simulink model "droneCorke"  (R2018a)
settings: Solver=VariableStepAuto  StartTime=0.0  StopTime=10.0  RelTol=1e-3
values from neighbouring files (symbols this model uses):
  MapMatrix = diag([ 1, -1, -1, -1, -1, 1, 1, -1, -1, -1, -1, 1])    [droneCorkeInit.m]
undefined symbols (not defined in the file or in its folder): Cofficients, quadrotor
libraries: simulink x14, roblocks x2
settings Model: Creator=dinies33  LastModifiedBy=dinies33

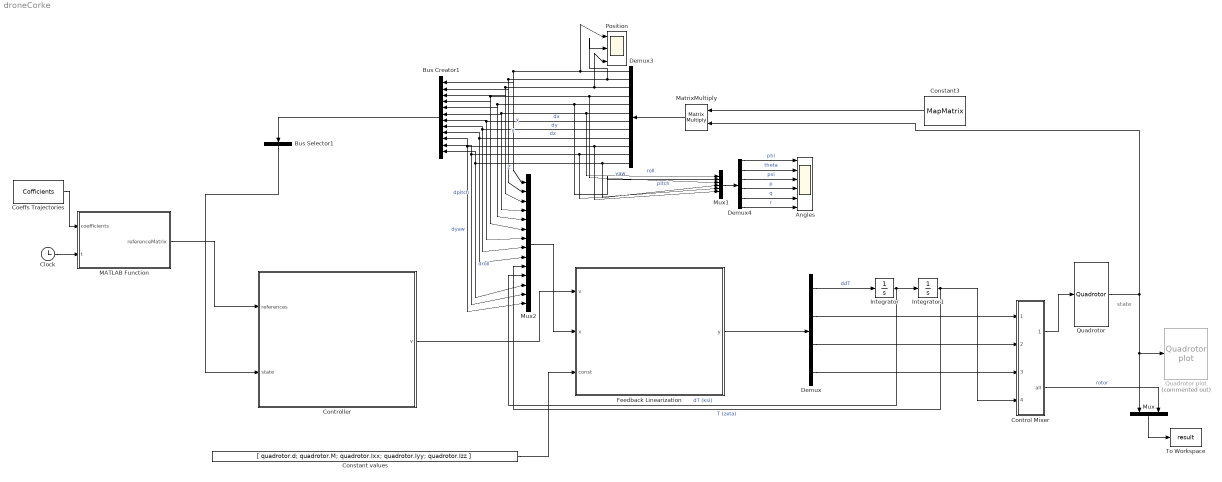
== system droneCorke ==
  note: state
  Angles : Scope  NumInputPorts=6
  Bus Creator1 : BusCreator  Inputs='X','Y','Z','yaw','pitch','roll','dx','dy','dz','dyaw','dpitch','droll'
  Bus Selector1 : BusSelector  OutputSignals=X,Y,Z,dx,dy,dz,yaw,dyaw  OutputAsBus=on
  Clock : Clock
  Coeffs Trajectories : Constant  Value=Cofficients
  Constant values : Constant  Value=[ quadrotor.d; quadrotor.M; quadrotor.Ixx; quadrotor.Iyy; quadrotor.Izz ]
  Constant3 : Constant  Value=MapMatrix
  Control Mixer : Subsystem  AncestorBlock=roblocks/Vehicles/Control Mixer 4  mask{quad=quadrotor, maxrot=1000, minrot=5}
      mask prompts: quad "Quadrotor parameters"; maxrot "Maximum rotor speed (rad/s)"; minrot "Minimum rotor speed (rad/s)"
      mask help: Quadrotor control mixer
      mask Help:
      | Determine rotor speeds based on desired torques and thrust, and propellor model
      | 
      | <b>Inputs::</b>
      | tau<sub>x</sub> (1x1)    desired rolling torque [Nm]
      | 
      | tau<sub>y</sub> (1x1)    desired pitching torque [Nm]
      | tau<sub>z</sub> (1x1)    desired yawing torque [Nm]
      | T (1x1)          desired thrust [N]
      | 
      | <b>Outputs::</b>
      | 
      | w1 (1x1) angular velocity of rotor 1 [rad]
      | w2 (1x1) angular velocity of rotor 2 [rad]
      | w3 (1x1) angular velocity of rotor 3 [rad]
      | w4 (1x1) angular velocity of rotor 4 [rad]
      | 
      | <b>Notes::</b>
      | 
      | - Assumes the rotor labelling convention of RVC Fig 4.16.
      | - The quadrotor is underactuated and has only 4 inputs.
      mask Display:
      | port_label('output',1,'\varpi','texmode','on');
      | port_label('output',2,'\tau_a','texmode','on');
      | port_label('input',1,'\tau_x','texmode','on');
      | port_label('input',2,'\tau_y','texmode','on');
      | port_label('input',3,'\tau_z','texmode','on');
      | port_label('input',4,'T','texmode','on');
  Controller : Subsystem
  Demux : Demux
  Demux3 : Demux  Outputs=12
  Demux4 : Demux  Outputs=6
  Feedback Linearization : MATLAB Function  TreatAsAtomicUnit=on
  Integrator : Integrator
  Integrator1 : Integrator
  MATLAB Function : MATLAB Function  TreatAsAtomicUnit=on
  MatrixMultiply : Product  Multiplication=Matrix(*)
  Mux : Mux  Inputs=2
  Mux1 : Mux  Inputs=6
  Mux2 : Mux  Inputs=14
  Position : Scope  NumInputPorts=3
  Quadrotor : roblocks/Vehicles/Quadrotor  quad=quadrotor  x0=[0 0 -5]  groundflag=on
      link override Dynamics: FunctionName=corke_dynamics
  Quadrotor plot : roblocks/Vehicles/Quadrotor plot  Commented=on  quad=quadrotor  xydim=2  zdim=10
      link override Plotter: FunctionName=corke_plot  Parameters=[xydim, zdim], 1, 1,quad
  To Workspace : ToWorkspace  VariableName=result  SampleTime=-1
  wires:
  Control Mixer/1(omega) -> Quadrotor/1
  Control Mixer/2(all) -> Mux/2  "rotor"
  Demux/2 -> Control Mixer/1(tau roll)
  Mux/1 -> To Workspace/1
  Demux/3 -> Control Mixer/2(tau pitch)
  Demux/4 -> Control Mixer/3(tau yaw)
  Bus Creator1/1 -> Bus Selector1/1
  Demux3/7 -> Mux2/7, Bus Creator1/7  "dx"
  Constant3/1 -> MatrixMultiply/1
  Demux3/10 -> Mux1/6, Mux2/14, Bus Creator1/10  "dyaw"
  Demux3/5 -> Mux1/2, Mux2/5, Bus Creator1/5  "pitch"
  Quadrotor/1 -> MatrixMultiply/2, Quadrotor plot/1, Mux/1
  Demux3/11 -> Mux1/5, Mux2/13, Bus Creator1/11  "dpitch"
  Demux3/9 -> Mux2/9, Bus Creator1/9  "dz"
  Demux3/12 -> Mux1/4, Mux2/12, Bus Creator1/12  "droll"
  Demux3/3 -> Position/3, Mux2/3, Bus Creator1/3  "Z"
  Demux3/4 -> Mux1/3, Mux2/6, Bus Creator1/4  "yaw"
  Demux3/8 -> Mux2/8, Bus Creator1/8  "dy"
  MatrixMultiply/1 -> Demux3/1
  Demux3/2 -> Position/2, Mux2/2, Bus Creator1/2  "Y"
  Demux3/6 -> Mux2/4, Bus Creator1/6, Mux1/1  "roll"
  Demux4/1 -> Angles/1  "phi"
  Demux4/4 -> Angles/4  "p"
  Demux4/3 -> Angles/3  "psi"
  Demux4/2 -> Angles/2  "theta"
  Demux4/5 -> Angles/5  "q"
  Demux4/6 -> Angles/6  "r"
  Mux1/1 -> Demux4/1
  Demux3/1 -> Position/1, Mux2/1, Bus Creator1/1  "X"
  Constant values/1 -> Feedback Linearization/3(const)
  Feedback Linearization/1(y) -> Demux/1
  Demux/1 -> Integrator/1  "ddT"
  Integrator/1 -> Mux2/11, Integrator1/1  "dT (ksi)"
  Integrator1/1 -> Mux2/10, Control Mixer/4(total thrust)  "T (zeta)"
  Mux2/1 -> Feedback Linearization/2(x)
  Controller/1(v) -> Feedback Linearization/1(v)
  MATLAB Function/1(referenceMatrix) -> Controller/1(references)
  Clock/1 -> MATLAB Function/2(t)
  Coeffs Trajectories/1 -> MATLAB Function/1(coefficients)
  Bus Selector1/1 -> Controller/2(state)

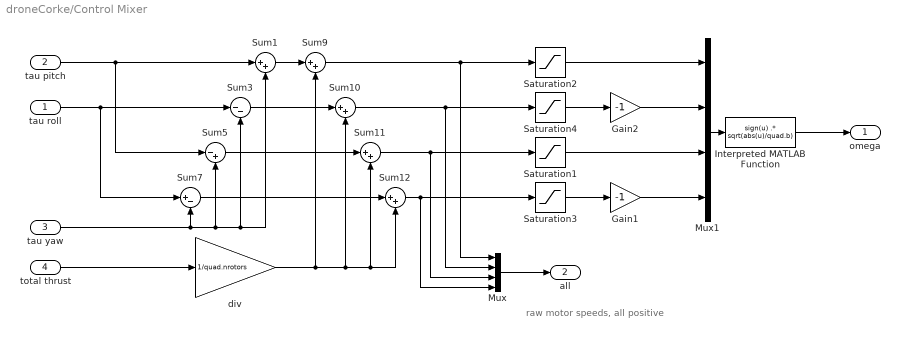
== system droneCorke/Control Mixer ==
  note: raw motor speeds, all positive
  tau roll : Inport
  tau pitch : Inport  Port=2
  tau yaw : Inport  Port=3
  total thrust : Inport  Port=4
  Gain1 : Gain  Gain=-1
  Gain2 : Gain  Gain=-1
  Interpreted MATLAB Function : MATLABFcn  MATLABFcn=sign(u) .* sqrt(abs(u)/quad.b)
  Mux : Mux
  Mux1 : Mux
  Saturation{1..4} (4 alike) : Saturate  UpperLimit=maxrot  LowerLimit=minrot
  Sum{1,9..12} (5 alike) : Sum  Inputs=|++  SaturateOnIntegerOverflow=on  InputSameDT=on  OutDataTypeStr=Inherit: Same as first input
  Sum3 : Sum  Inputs=|--  SaturateOnIntegerOverflow=on  InputSameDT=on  OutDataTypeStr=Inherit: Same as first input
  Sum5 : Sum  Inputs=|-+  SaturateOnIntegerOverflow=on  InputSameDT=on  OutDataTypeStr=Inherit: Same as first input
  Sum7 : Sum  Inputs=|+-  SaturateOnIntegerOverflow=on  InputSameDT=on  OutDataTypeStr=Inherit: Same as first input
  div : Gain  Gain=1/quad.nrotors
  omega : Outport
  all : Outport  Port=2
  wires:
  div/1 -> Sum11/2, Sum12/2, Sum10/2, Sum9/2
  Interpreted MATLAB Function/1 -> omega/1
  Mux1/1 -> Interpreted MATLAB Function/1
  tau yaw/1 -> Sum7/2, Sum5/2, Sum3/2, Sum1/2
  Saturation2/1 -> Mux1/1
  Saturation4/1 -> Gain2/1
  Saturation1/1 -> Mux1/3
  Saturation3/1 -> Gain1/1
  tau pitch/1 -> Sum1/1, Sum5/1
  Sum1/1 -> Sum9/1
  Sum3/1 -> Sum10/1
  Sum5/1 -> Sum11/1
  Sum7/1 -> Sum12/1
  Sum9/1 -> Saturation2/1, Mux/1
  Sum10/1 -> Mux/2, Saturation4/1
  Sum11/1 -> Mux/3, Saturation1/1
  Sum12/1 -> Mux/4, Saturation3/1
  total thrust/1 -> div/1
  tau roll/1 -> Sum3/1, Sum7/1
  Mux/1 -> all/1
  Gain1/1 -> Mux1/4
  Gain2/1 -> Mux1/2

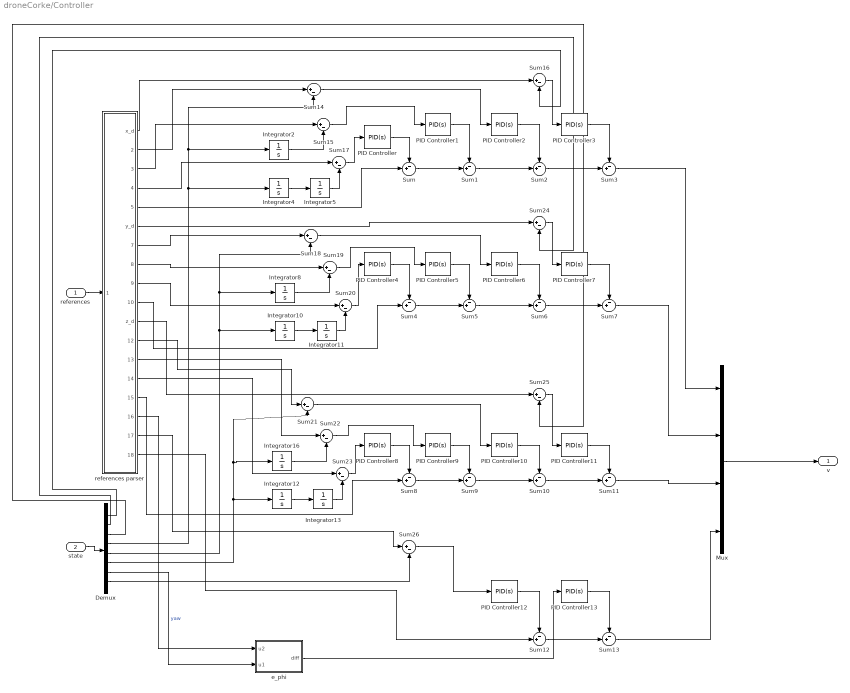
== system droneCorke/Controller ==
  references : Inport
  state : Inport  Port=2
  Demux : Demux  Outputs=8
  Integrator{2,4..5,8,10..13,16} (9 alike) : Integrator
  Mux : Mux
  PID Controller{,1..13} (14 alike) : simulink/Continuous/PID Controller  Controller=PID  TimeDomain=Continuous-time  SampleTime=-1  IntegratorMethod=Forward Euler  FilterMethod=Forward Euler  Form=Parallel  UseFilter=on  ControllerParametersSource=internal  P=1  I=1  D=0  N=100  InitialConditionSource=internal  InitialConditionForIntegrator=0  InitialConditionForFilter=0  ExternalReset=none  LimitOutput=off  UpperSaturationLimit=inf  LowerSaturationLimit=-inf  LinearizeAsGain=on  AntiWindupMode=none  Kb=1  TrackingMode=off  Kt=1  PParamMin=[]  PParamMax=[]  IParamMin=[]  IParamMax=[]  DParamMin=[]  DParamMax=[]  NParamMin=[]  NParamMax=[]  KbParamMin=[]  KbParamMax=[]  KtParamMin=[]  KtParamMax=[]  POutMin=[]  POutMax=[]  IOutMin=[]  IOutMax=[]  DOutMin=[]  DOutMax=[]  NOutMin=[]  NOutMax=[]  KbOutMin=[]  KbOutMax=[]  KtOutMin=[]  KtOutMax=[]  IntegratorOutMin=[]  IntegratorOutMax=[]  FilterOutMin=[]  FilterOutMax=[]  SumOutMin=[]  SumOutMax=[]  SumI1OutMin=[]  SumI1OutMax=[]  SumI2OutMin=[]  SumI2OutMax=[]  SumI3OutMin=[]  SumI3OutMax=[]  SumDOutMin=[]  SumDOutMax=[]  SaturationOutMin=[]  SaturationOutMax=[]  IntegratorContinuousStateAttributes=''  IntegratorStateMustResolveToSignalObject=off  IntegratorRTWStateStorageClass=Auto  FilterContinuousStateAttributes=''  FilterStateMustResolveToSignalObject=off  FilterRTWStateStorageClass=Auto  DifferentiatorICPrevScaledInput=0  DifferentiatorOutMin=[]  DifferentiatorOutMax=[]  FilterDiffOutCoefMin=[]  FilterDiffOutCoefMax=[]  SumDenOutMin=[]  SumDenOutMax=[]  SumNumOutMin=[]  SumNumOutMax=[]  ReciprocalOutMin=[]  ReciprocalOutMax=[]  DivideOutMin=[]  DivideOutMax=[]  TunerSelectOption=Transfer Function Based (PID Tuner App)
  Sum{,1..13} (14 alike) : Sum  Inputs=-+|
  Sum{14..26} (13 alike) : Sum  Inputs=|+-
  e_phi : MATLAB Function  TreatAsAtomicUnit=on
  references parser : MATLAB Function  TreatAsAtomicUnit=on
  v : Outport
  wires:
  Sum3/1 -> Mux/1
  Sum7/1 -> Mux/2
  Mux/1 -> v/1
  Sum11/1 -> Mux/3
  Sum13/1 -> Mux/4
  PID Controller11/1 -> Sum11/1
  Sum10/1 -> Sum11/2
  PID Controller10/1 -> Sum10/1
  Sum9/1 -> Sum10/2
  PID Controller9/1 -> Sum9/1
  Sum8/1 -> Sum9/2
  PID Controller8/1 -> Sum8/1
  PID Controller4/1 -> Sum4/1
  Sum4/1 -> Sum5/2
  PID Controller5/1 -> Sum5/1
  Sum5/1 -> Sum6/2
  PID Controller6/1 -> Sum6/1
  Sum6/1 -> Sum7/2
  PID Controller7/1 -> Sum7/1
  PID Controller3/1 -> Sum3/1
  Sum2/1 -> Sum3/2
  PID Controller2/1 -> Sum2/1
  Sum1/1 -> Sum2/2
  PID Controller1/1 -> Sum1/1
  Sum/1 -> Sum1/2
  PID Controller/1 -> Sum/1
  PID Controller12/1 -> Sum12/1
  PID Controller13/1 -> Sum13/1
  Sum12/1 -> Sum13/2
  references/1 -> references parser/1(matrix)
  references parser/16(psi_d) -> e_phi/1(u2)
  e_phi/1(diff) -> PID Controller13/1
  state/1 -> Demux/1
  Demux/7 -> e_phi/2(u1)  "yaw"
  Demux/4 -> Integrator4/1, Sum14/2, Integrator2/1
  references parser/1(x_d) -> Sum16/1
  Sum16/1 -> PID Controller3/1
  Sum14/1 -> PID Controller2/1
  references parser/5(ddddx_d) -> Sum/2
  Sum15/1 -> PID Controller1/1
  Integrator2/1 -> Sum15/2
  Integrator4/1 -> Integrator5/1
  references parser/4(dddx_d) -> Sum17/1
  Integrator5/1 -> Sum17/2
  Sum17/1 -> PID Controller/1
  references parser/2(dx_d) -> Sum14/1
  references parser/3(ddx_d) -> Sum15/1
  Demux/5 -> Integrator10/1, Sum18/2, Integrator8/1
  Integrator11/1 -> Sum20/2
  Integrator10/1 -> Integrator11/1
  Integrator8/1 -> Sum19/2
  Demux/6 -> Integrator12/1, Integrator16/1, Sum21/2
  Integrator13/1 -> Sum23/2
  Integrator12/1 -> Integrator13/1
  Integrator16/1 -> Sum22/2
  references parser/6(y_d) -> Sum24/1
  references parser/7(dy_d) -> Sum18/1
  references parser/8(ddy_d) -> Sum19/1
  references parser/9(dddy_d) -> Sum20/1
  Demux/1 -> Sum16/2
  Demux/2 -> Sum24/2
  Demux/3 -> Sum25/2
  Sum25/1 -> PID Controller11/1
  Sum24/1 -> PID Controller7/1
  references parser/11(z_d) -> Sum25/1
  Sum18/1 -> PID Controller6/1
  Sum19/1 -> PID Controller5/1
  Sum20/1 -> PID Controller4/1
  references parser/15(ddddz_d) -> Sum8/2
  references parser/10(ddddy_d) -> Sum4/2
  references parser/12(dz_d) -> Sum21/1
  references parser/13(ddz_d) -> Sum22/1
  references parser/14(dddz_d) -> Sum23/1
  Sum21/1 -> PID Controller10/1
  Sum22/1 -> PID Controller9/1
  Sum23/1 -> PID Controller8/1
  references parser/18(ddpsi_d) -> Sum12/2
  Demux/8 -> Sum26/2
  references parser/17(dpsi_d) -> Sum26/1
  Sum26/1 -> PID Controller12/1

== matlab function droneCorke/MATLAB Function ==
  data: coefficients input; t input; referenceMatrix output
function referenceMatrix = fcn(coefficients,t)
referenceMatrix = zeros(5,4);

for i = 1:size(coefficients,2)
    a = self.coefficients(1,i);
    b = self.coefficients(2,i);
    c = self.coefficients(3,i);
    d = self.coefficients(4,i);
    e = self.coefficients(5,i);
    f = self.coefficients(6,i);
    g = self.coefficients(7,i);
    h = self.coefficients(8,i);
    m = self.coefficients(9,i);
    l = self.coefficients(10,i);
    poly = @(t) [
        a*t^9     + b*t^8      + c*t^7      + d*t^6     + e*t^5    + f*t^4    + g*t^3   + h*t^2 + m*t + l ;
        9*a*t^8   + 8*b*t^7    + 7*c*t^6    + 6*d*t^5   + 5*e*t^4  + 4*f*t^3  + 3*g*t^2 + 2*h*t + m       ;
        72*a*t^7  + 56*b*t^6   + 42*c*t^5   + 30*d*t^4  + 20*e*t^3 + 12*f*t^2 + 6*g*t   + 2*h             ;
        504*a*t^6 + 336*b*t^5  + 210*c*t^4  + 120*d*t^3 + 60*e*t^2 + 24*f*t   + 6*g                       ;
        3024*a*t^5+ 1680*b*t^4 + 840*c*t^3  + 360*d*t^2 + 120*e*t  + 24*f
        ];
    eval = poly(t);
    
    referenceMatrix(1,i)= eval(1,1);
    referenceMatrix(2,i)= eval(2,1);
    referenceMatrix(3,i)= eval(3,1);
    referenceMatrix(4,i)= eval(4,1);
    referenceMatrix(5,i)= eval(5,1);
    
end
end

== matlab function droneCorke/Feedback Linearization ==
  data: v input; y output; x input; const input
function y = fcn(v,x,const)

d= constants(1,1);
M= constants(2,1);
I_1= constants(3,1);
I_2= constants(4,1);
I_3= constants(5,1);


% q1 = x(1,1);
% q2 = x(2,1);
% q3 = x(3,1);
q4 = x(4,1);
q5 = x(5,1);
q6 = x(6,1);
q10 = x(10,1);
q11 = x(11,1);
q12 = x(12,1);
q13 = x(13,1);
q14 = x(14,1);


delta = zeros(4,4);

delta(1,:)=  [ -(sin(q4)*sin(q6) + cos(q4)*cos(q6)*sin(q5))/M, -(d*q10*(cos(q4)*sin(q6) - cos(q6)*sin(q4)*sin(q5)))/(I_1*M), -(d*q10*cos(q4)*cos(q5)*cos(q6))/(I_2*M), -(q10*(cos(q6)*sin(q4) - cos(q4)*sin(q5)*sin(q6)))/(I_3*M)];


delta(2,:)=  [  (cos(q6)*sin(q4) - cos(q4)*sin(q5)*sin(q6))/M,  (d*q10*(cos(q4)*cos(q6) + sin(q4)*sin(q5)*sin(q6)))/(I_1*M), -(d*q10*cos(q4)*cos(q5)*sin(q6))/(I_2*M), -(q10*(sin(q4)*sin(q6) + cos(q4)*cos(q6)*sin(q5)))/(I_3*M)];


delta(3,:)= [ -(cos(q4)*cos(q5))/M, (d*q10*cos(q5)*sin(q4))/(I_1*M), (d*q10*cos(q4)*sin(q5))/(I_2*M),  0];

delta(4,:)= [   0, 0,  0,  1/I_3];





bVec = zeros(4,1);

bVec(1,1) =  q13*((q10*q12*cos(q5)*cos(q6)*sin(q4))/M - (q11*cos(q4)*cos(q5)*cos(q6))/M + (q10*q13*cos(q4)*cos(q6)*sin(q5))/M + (q10*q14*cos(q4)*cos(q5)*sin(q6))/M) - q12*((q11*(cos(q4)*sin(q6) - cos(q6)*sin(q4)*sin(q5)))/M - (q10*q12*(sin(q4)*sin(q6) + cos(q4)*cos(q6)*sin(q5)))/M + (q10*q14*(cos(q4)*cos(q6) + sin(q4)*sin(q5)*sin(q6)))/M - (q10*q13*cos(q5)*cos(q6)*sin(q4))/M) - q14*((q11*(cos(q6)*sin(q4) - cos(q4)*sin(q5)*sin(q6)))/M + (q10*q12*(cos(q4)*cos(q6) + sin(q4)*sin(q5)*sin(q6)))/M - (q10*q14*(sin(q4)*sin(q6) + cos(q4)*cos(q6)*sin(q5)))/M - (q10*q13*cos(q4)*cos(q5)*sin(q6))/M) - q11*((q12*(cos(q4)*sin(q6) - cos(q6)*sin(q4)*sin(q5)))/M + (q14*(cos(q6)*sin(q4) - cos(q4)*sin(q5)*sin(q6)))/M + (q13*cos(q4)*cos(q5)*cos(q6))/M) - (q10*q12*q13*(I_1 - I_2)*(cos(q6)*sin(q4) - cos(q4)*sin(q5)*sin(q6)))/(I_3*M) - (q10*q13*q14*(I_2 - I_3)*(cos(q4)*sin(q6) - cos(q6)*sin(q4)*sin(q5)))/(I_1*M) + (q10*q12*q14*cos(q4)*cos(q5)*cos(q6)*(I_1 - I_3))/(I_2*M);



bVec(2,1) =  q12*((q11*(cos(q4)*cos(q6) + sin(q4)*sin(q5)*sin(q6)))/M - (q10*q12*(cos(q6)*sin(q4) - cos(q4)*sin(q5)*sin(q6)))/M - (q10*q14*(cos(q4)*sin(q6) - cos(q6)*sin(q4)*sin(q5)))/M + (q10*q13*cos(q5)*sin(q4)*sin(q6))/M) - q14*((q11*(sin(q4)*sin(q6) + cos(q4)*cos(q6)*sin(q5)))/M + (q10*q12*(cos(q4)*sin(q6) - cos(q6)*sin(q4)*sin(q5)))/M + (q10*q14*(cos(q6)*sin(q4) - cos(q4)*sin(q5)*sin(q6)))/M + (q10*q13*cos(q4)*cos(q5)*cos(q6))/M) - q11*((q14*(sin(q4)*sin(q6) + cos(q4)*cos(q6)*sin(q5)))/M - (q12*(cos(q4)*cos(q6) + sin(q4)*sin(q5)*sin(q6)))/M + (q13*cos(q4)*cos(q5)*sin(q6))/M) - q13*((q11*cos(q4)*cos(q5)*sin(q6))/M + (q10*q14*cos(q4)*cos(q5)*cos(q6))/M - (q10*q12*cos(q5)*sin(q4)*sin(q6))/M - (q10*q13*cos(q4)*sin(q5)*sin(q6))/M) - (q10*q12*q13*(I_1 - I_2)*(sin(q4)*sin(q6) + cos(q4)*cos(q6)*sin(q5)))/(I_3*M) + (q10*q13*q14*(I_2 - I_3)*(cos(q4)*cos(q6) + sin(q4)*sin(q5)*sin(q6)))/(I_1*M) + (q10*q12*q14*cos(q4)*cos(q5)*sin(q6)*(I_1 - I_3))/(I_2*M);



bVec(3,1) =  q11*((q12*cos(q5)*sin(q4))/M + (q13*cos(q4)*sin(q5))/M) + q12*((q11*cos(q5)*sin(q4))/M + (q10*q12*cos(q4)*cos(q5))/M - (q10*q13*sin(q4)*sin(q5))/M) + q13*((q11*cos(q4)*sin(q5))/M + (q10*q13*cos(q4)*cos(q5))/M - (q10*q12*sin(q4)*sin(q5))/M) - (q10*q12*q14*cos(q4)*sin(q5)*(I_1 - I_3))/(I_2*M) + (q10*q13*q14*cos(q5)*sin(q4)*(I_2 - I_3))/(I_1*M);


bVec(4,1) = (q12*q13*(I_1 - I_2))/I_3;



invDelta = inv(delta + 3.5*eye(4));  %TODO remove regularization
alfa = - invDelta * bVec;
beta = invDelta;
y = alfa + beta * v;

== matlab function droneCorke/Controller/references parser ==
  data: matrix input; x_d output; dx_d output; ddx_d output; dddx_d output; ddddx_d output; y_d output; dy_d output; ddy_d output; dddy_d output; ddddy_d output; z_d output; dz_d output; ddz_d output; dddz_d output; ddddz_d output; psi_d output; dpsi_d output; ddpsi_d output
function [x_d,dx_d,ddx_d,dddx_d,ddddx_d,y_d,dy_d,ddy_d,dddy_d,ddddy_d,z_d,dz_d,ddz_d,dddz_d,ddddz_d,psi_d,dpsi_d,ddpsi_d] = fcn(matrix)
x_d = matrix(1,1);
dx_d = matrix(2,1);
ddx_d = matrix(3,1);
dddx_d = matrix(4,1);
ddddx_d = matrix(5,1);
y_d = matrix(1,2);
dy_d = matrix(2,2);
ddy_d = matrix(3,2);
dddy_d = matrix(4,2);
ddddy_d = matrix(5,2);
z_d = matrix(1,3);
dz_d = matrix(2,3);
ddz_d = matrix(3,3);
dddz_d = matrix(4,3);
ddddz_d = matrix(5,3);
psi_d = matrix(1,4);
dpsi_d = matrix(2,4);
ddpsi_d = matrix(3,4);

== matlab function droneCorke/Controller/e_phi ==
  data: u2 input; diff output; u1 input
function diff = fcn(u2, u1)

R2 = [cos(u2) -sin(u2);
      sin(u2) cos(u2)];

R1 = [cos(-u1) -sin(-u1);
      sin(-u1) cos(-u1)];

R = R2*R1;

diff = atan2(R(2,1), R(1,1));
